simulink model "ff_test_simple"  (R2023b)
settings: Solver=VariableStepAuto  StartTime=0.0  StopTime=10  RelTol=1e-3
values from neighbouring files (symbols this model uses):
  D = 0.000001    (= 1e-06)    [motor_param.m]
  g = 1    [motor_param.m]
  J = 0.151e-7    (= 1.51e-08)    [motor_param.m]
  K_e = 1    [ff_inv.m]    (also in motor_param.m = 0.00352372567731)
  K_t = 1    [ff_inv.m]    (also in motor_param.m = 0.00352)
  L = 0.045    [motor_param.m]
  m = 1    [ff_inv.m]    (also in motor_param.m = 0.15)
  R = 1    [ff_inv.m]    (also in motor_param.m = 2.9)
  r = 1    [ff_inv.m]    (also in motor_param.m = 0.012)
settings Model: Creator=under  LastModifiedBy=under

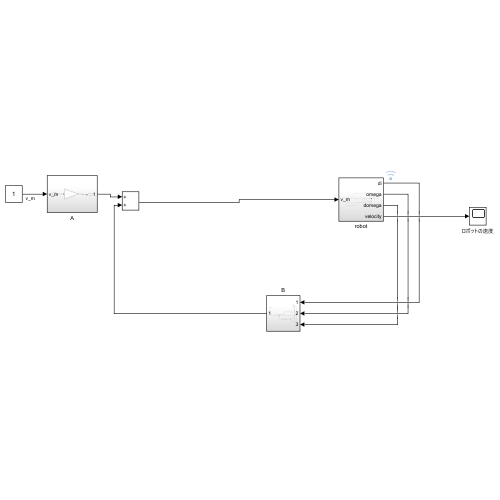
[thumbnail: Simulink's stored preview of the top-level diagram]
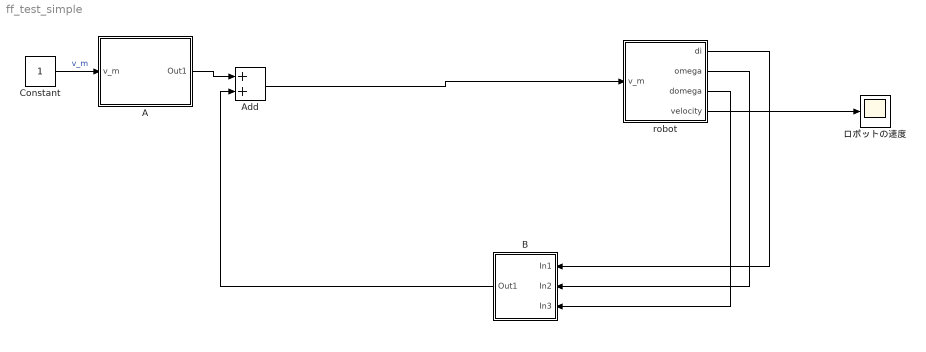
== system ff_test_simple ==
  A : Subsystem
  Add : Sum
  B : Subsystem
  Constant : Constant
  robot : Subsystem
  ロボットの速度 : Scope
  wires:
  robot/4(velocity) -> ロボットの速度/1
  Add/1 -> robot/1(v_m)
  Constant/1 -> A/1(v_m)  "v_m"
  A/1(Out1) -> Add/1
  robot/1(di) -> B/1(In1)
  robot/2(omega) -> B/2(In2)
  robot/3(domega) -> B/3(In3)
  B/1(Out1) -> Add/2

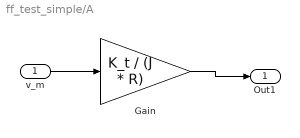
== system ff_test_simple/A ==
  v_m : Inport
  Gain : Gain  Gain=K_t / (J * R)
  Out1 : Outport
  wires:
  v_m/1 -> Gain/1
  Gain/1 -> Out1/1

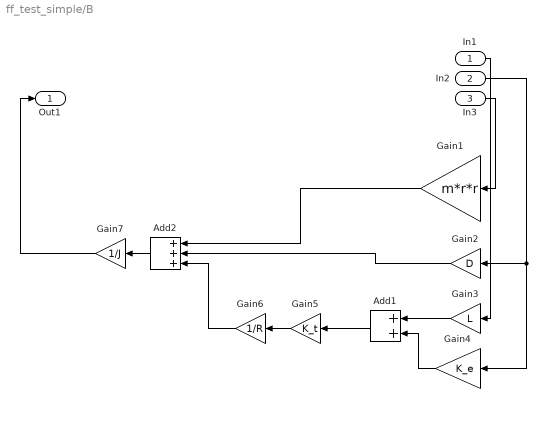
== system ff_test_simple/B ==
  In1 : Inport
  In2 : Inport  Port=2
  In3 : Inport  Port=3
  Add1 : Sum
  Add2 : Sum  Inputs=+++
  Gain1 : Gain  Gain=m*r*r
  Gain2 : Gain  Gain=D
  Gain3 : Gain  Gain=L
  Gain4 : Gain  Gain=K_e
  Gain5 : Gain  Gain=K_t
  Gain6 : Gain  Gain=1/R
  Gain7 : Gain  Gain=1/J
  Out1 : Outport
  wires:
  Gain1/1 -> Add2/1
  Add1/1 -> Gain5/1
  Gain2/1 -> Add2/2
  Gain5/1 -> Gain6/1
  Gain3/1 -> Add1/1
  Gain4/1 -> Add1/2
  In2/1 -> Gain4/1, Gain2/1
  Gain7/1 -> Out1/1
  Gain6/1 -> Add2/3
  In3/1 -> Gain1/1
  Add2/1 -> Gain7/1
  In1/1 -> Gain3/1

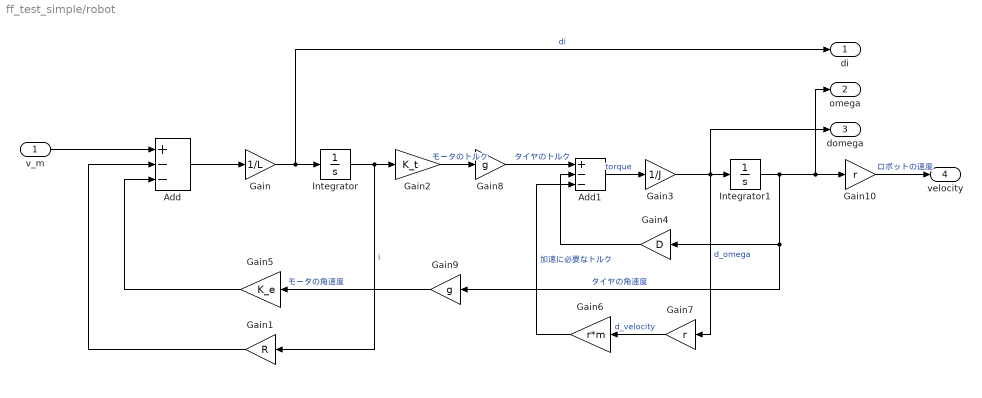
== system ff_test_simple/robot ==
  v_m : Inport
  Add : Sum  Inputs=+--
  Add1 : Sum  Inputs=+--
  Gain : Gain  Gain=1/L
  Gain1 : Gain  Gain=R
  Gain10 : Gain  Gain=r
  Gain2 : Gain  Gain=K_t
  Gain3 : Gain  Gain=1/J
  Gain4 : Gain  Gain=D
  Gain5 : Gain  Gain=K_e
  Gain6 : Gain  Gain=r*m
  Gain7 : Gain  Gain=r
  Gain8 : Gain  Gain=g
  Gain9 : Gain  Gain=g
  Integrator : Integrator
  Integrator1 : Integrator
  di : Outport
  omega : Outport  Port=2
  domega : Outport  Port=3
  velocity : Outport  Port=4
  wires:
  Gain5/1 -> Add/3
  Gain2/1 -> Gain8/1  "モータのトルク"
  Gain3/1 -> Integrator1/1, domega/1, Gain7/1  "d_omega"
  Integrator/1 -> Gain2/1, Gain1/1  "i"
  Gain1/1 -> Add/2
  Gain/1 -> di/1, Integrator/1  "di"
  Add/1 -> Gain/1
  Integrator1/1 -> omega/1, Gain10/1, Gain4/1, Gain9/1  "タイヤの角速度"
  Add1/1 -> Gain3/1  "torque"
  Gain4/1 -> Add1/2
  v_m/1 -> Add/1
  Gain6/1 -> Add1/3  "加速に必要なトルク"
  Gain7/1 -> Gain6/1  "d_velocity"
  Gain8/1 -> Add1/1  "タイヤのトルク"
  Gain9/1 -> Gain5/1  "モータの角速度"
  Gain10/1 -> velocity/1  "ロボットの速度"
